simulink model "tan_blf"  (R2021a)
settings: Solver=VariableStepAuto  StartTime=0.0  StopTime=10  RelTol=1e-3
settings Model: Creator=28355  LastModifiedBy=28355

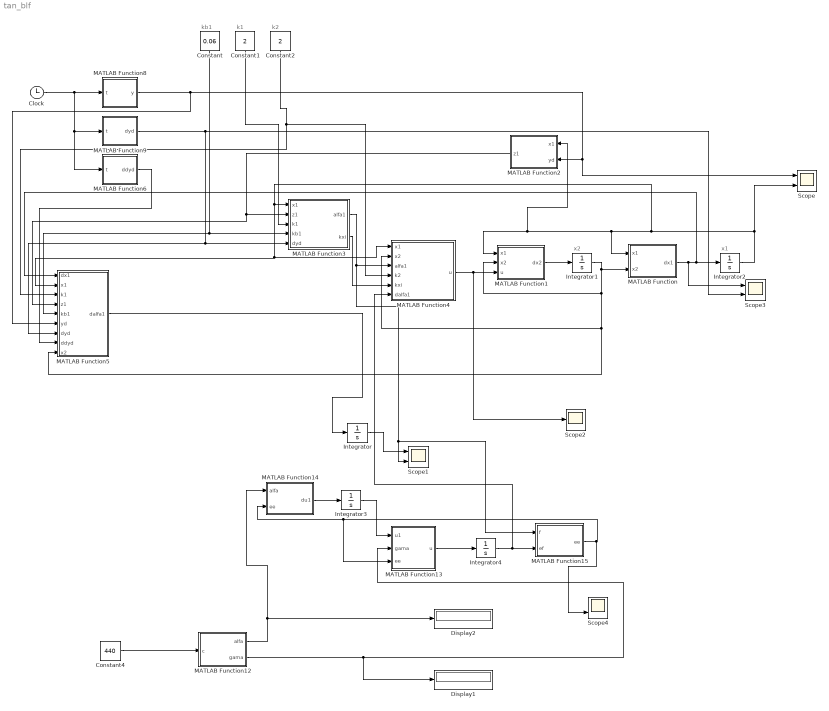
== system tan_blf ==
  note: x2
  note: x1
  note: k1
  note: kb1
  note: k2
  Clock : Clock
  Constant : Constant  Value=0.06
  Constant1 : Constant  Value=2
  Constant2 : Constant  Value=2
  Constant4 : Constant  Value=440
  Display1 : Display
  Display2 : Display
  Integrator : Integrator
  Integrator1 : Integrator  InitialCondition=1.5
  Integrator2 : Integrator  InitialCondition=0.25
  Integrator3 : Integrator
  Integrator4 : Integrator  InitialCondition=1
  MATLAB Function : MATLAB Function  TreatAsAtomicUnit=on
  MATLAB Function1 : MATLAB Function  TreatAsAtomicUnit=on
  MATLAB Function12 : MATLAB Function  TreatAsAtomicUnit=on
  MATLAB Function13 : MATLAB Function  TreatAsAtomicUnit=on
  MATLAB Function14 : MATLAB Function  TreatAsAtomicUnit=on
  MATLAB Function15 : MATLAB Function  TreatAsAtomicUnit=on
  MATLAB Function2 : MATLAB Function  TreatAsAtomicUnit=on
  MATLAB Function3 : MATLAB Function  TreatAsAtomicUnit=on
  MATLAB Function4 : MATLAB Function  TreatAsAtomicUnit=on
  MATLAB Function5 : MATLAB Function  TreatAsAtomicUnit=on
  MATLAB Function6 : MATLAB Function  TreatAsAtomicUnit=on
  MATLAB Function8 : MATLAB Function  TreatAsAtomicUnit=on
  MATLAB Function9 : MATLAB Function  TreatAsAtomicUnit=on
  Scope{,1,3..4} (4 alike) : Scope  NumInputPorts=2
  Scope2 : Scope
  wires:
  MATLAB Function/1(dx1) -> Scope3/1, MATLAB Function5/1(dx1), Integrator2/1
  Integrator1/1 -> MATLAB Function4/2(x2), MATLAB Function5/9(x2), MATLAB Function1/2(x2), MATLAB Function/2(x2)
  MATLAB Function1/1(dx2) -> Integrator1/1
  Clock/1 -> MATLAB Function6/1(t), MATLAB Function9/1(t), MATLAB Function8/1(t)
  MATLAB Function4/1(u) -> Scope2/1, MATLAB Function1/3(u)
  MATLAB Function8/1(y) -> MATLAB Function5/6(yd), Scope/1, MATLAB Function2/2(yd)
  MATLAB Function2/1(z1) -> MATLAB Function3/2(z1), MATLAB Function5/4(z1)
  Integrator2/1 -> Scope/2, MATLAB Function5/2(x1), MATLAB Function4/1(x1), MATLAB Function3/1(x1), MATLAB Function1/1(x1), MATLAB Function2/1(x1), MATLAB Function/1(x1)
  MATLAB Function9/1(dyd) -> Scope3/2, MATLAB Function5/7(dyd), MATLAB Function3/5(dyd)
  MATLAB Function6/1(ddyd) -> MATLAB Function5/8(ddyd)
  MATLAB Function5/1(dalfa1) -> Integrator/1
  MATLAB Function3/1(alfa1) -> MATLAB Function15/1(f), Scope1/2, MATLAB Function4/3(alfa1)
  Constant/1 -> MATLAB Function3/4(kb1), MATLAB Function5/5(kb1)
  Constant1/1 -> MATLAB Function3/3(k1)
  Constant2/1 -> MATLAB Function4/4(k2), MATLAB Function5/3(k1)
  MATLAB Function3/2(kxi) -> MATLAB Function4/5(kxi)
  Integrator/1 -> Scope1/1
  MATLAB Function15/1(ee) -> Scope4/2, MATLAB Function13/3(ee), MATLAB Function14/2(ee)
  Integrator4/1 -> MATLAB Function4/6(dalfa1), MATLAB Function15/2(ef)
  Constant4/1 -> MATLAB Function12/1(c)
  MATLAB Function12/2(gama) -> Display1/1, MATLAB Function13/2(gama)
  MATLAB Function12/1(alfa) -> Display2/1, MATLAB Function14/1(alfa)
  Integrator3/1 -> MATLAB Function13/1(u1)
  MATLAB Function13/1(u) -> Integrator4/1
  MATLAB Function14/1(du1) -> Integrator3/1

== matlab function tan_blf/MATLAB Function12 ==
  data: c input; alfa output; gama output
function [alfa, gama] = fcn(c)

alfa = ceil(4 * c);
gama = ceil(sqrt(20 * c / 3));

== matlab function tan_blf/MATLAB Function13 ==
  data: u1 input; u output; gama input; ee input
function u = fcn(u1, gama, ee)

u = u1 - gama * (abs(ee))^0.5*sign(ee);

== matlab function tan_blf/MATLAB Function14 ==
  data: alfa input; du1 output; ee input
function du1 = fcn(alfa, ee)

du1 = -alfa*sign(ee);

== matlab function tan_blf/MATLAB Function15 ==
  data: f input; ee output; ef input
function ee = fcn(f, ef)

ee = ef - f;

== matlab function tan_blf/MATLAB Function1 ==
  data: x1 input; x2 input; u input; dx2 output
function dx2 = fcn(x1, x2, u)

dx2 = 0.1 * x1 * x2 - 0.2 * x1 + (1 + x1^2) * u;

== matlab function tan_blf/MATLAB Function ==
  data: x1 input; dx1 output; x2 input
function dx1 = fcn( x1,x2)

dx1= 0.1 * x1^2 + x2;

== matlab function tan_blf/MATLAB Function2 ==
  data: x1 input; z1 output; yd input
function z1 = fcn(x1, yd)

z1 = x1 - yd;

== matlab function tan_blf/MATLAB Function3 ==
  data: x1 input; alfa1 output; z1 input; k1 input; kb1 input; dyd input; kxi output
function [alfa1,kxi]  = fcn(x1, z1, k1, kb1, dyd)

kxi = pi * z1 / (2 * kb1);
alfa1 = - 0.1 * x1^2 - k1 * z1^2 * (cos(kxi))^3 / sin(kxi) + dyd;

== matlab function tan_blf/MATLAB Function4 ==
  data: x1 input; u output; x2 input; alfa1 input; k2 input; kxi input; dalfa1 input
function u = fcn(x1, x2, alfa1, k2, kxi, dalfa1)

z2 = x2 - alfa1;
g2 = 1 + x1^2;
f2 = 0.1 * x1 * x2 - 0.2 * x2;
u = (- f2 + dalfa1 - k2 * z2 - sin(kxi)/(cos(kxi))^3)/g2;

== matlab function tan_blf/MATLAB Function5 ==
  data: dx1 input; dalfa1 output; x1 input; k1 input; z1 input; kb1 input; yd input; dyd input; ddyd input; x2 input
function dalfa1 = fcn(dx1, x1, k1, z1, kb1,yd, dyd, ddyd, x2)

f1 = 0.1 * x1^2;
kxi = pi * z1 / (2 * kb1);
kxi_x = pi * dx1 / (2 * kb1);
dalfa1_x1 = - 0.2 * x1 * dx1 + k1 * z1^2 * (cos(kxi))^4 / (sin(kxi))^2 * kxi_x - ...
    2 * k1 * z1 * dx1 * (cos(kxi))^3 / sin(kxi) + 3 * k1 * z1^2 *...
    (cos(kxi))^2 * kxi_x;
dalfa1_yd = ddyd / dyd;
dalfa1 = dalfa1_x1 * (f1 + x2) + dalfa1_yd * yd^2;

== matlab function tan_blf/MATLAB Function6 ==
  data: t input; ddyd output
function ddyd = fcn(t)

ddyd = - 0.3 * sin(t);

== matlab function tan_blf/MATLAB Function8 ==
  data: t input; y output
function y = fcn(t)

y = 0.2 + 0.3 * sin(t);

== matlab function tan_blf/MATLAB Function9 ==
  data: t input; dyd output
function dyd = fcn(t)

dyd = 0.3 * cos(t);
